simulink model "MPC_Shell3x3"  (R2021a)
settings: Solver=FixedStepAuto  StartTime=0  StopTime=1999  FixedStep=Ts  RelTol=1e-3
undefined symbols (not defined in the file or in its folder): L, R
libraries: simulink x3, mpclib x1, cstblocks x1
settings Model: Creator=Sergio Castaño  LastModifiedBy=Sergio
settings SolverCC: AlgebraicLoopSolver=TrustRegion
settings DataIOCC: LimitDataPoints=on  ReturnWorkspaceOutputs=off
settings OptimizationCC: DefaultParameterBehavior=Inlined  UseFloatMulNetSlope=on  InlineInvariantSignals=on  EnhancedBackFolding=on  PassReuseOutputArgsAs=Individual arguments  EfficientFloat2IntCast=on  LifeSpan=inf  EfficientTunableParamExpr=on
settings DebuggingCC: ParameterTunabilityLossMsg=error  AllowSymbolicDim=off  SFUnexpectedBacktrackingDiag=warning  SFNoUnconditionalDefaultTransitionDiag=warning  SFExecutionAtInitializationDiag=none  SFMachineParentedDataDiag=warning  ArithmeticOperatorsInVariantConditions=warning
settings HardwareCC: ProdBitPerSizeT=32  ProdBitPerPtrDiffT=32  ProdWordSize=32  ProdHWDeviceType=Specified
settings ModelReferenceCC: UpdateModelReferenceTargets=AssumeUpToDate  CheckModelReferenceTargetMessage=none  EnableParallelModelReferenceBuilds=on  PropagateSignalLabelsOutOfModel=off
settings SFSimCC: SimUseLocalCustomCode=off  MATLABDynamicMemAlloc=off  CustomCodeUndefinedFunction=UseInterfaceOnly
settings RTWCC: SystemTargetFile=ert.tlc  TemplateMakefile=ert_default_tmf  GenerateReport=on  RTWUseLocalCustomCode=off  IncludeHyperlinkInReport=on  LaunchReport=on  GenerateTraceInfo=on  GenerateTraceReport=on  GenerateTraceReportSl=on  GenerateTraceReportSf=on  GenerateTraceReportEml=on
settings CodeAppCC: ForceParamTrailComments=on  IgnoreCustomStorageClasses=off  OperatorAnnotations=on  SimulinkDataObjDesc=on  SFDataObjDesc=on  InsertBlockDesc=on  StateflowObjectComments=on
settings ERTTargetCC: GenerateSampleERTMain=on  SupportContinuousTime=on  InlinedParameterPlacement=NonHierarchical  ERTCustomFileTemplate=example_file_process.tlc
settings ConfigComp: CovMetricSettings=dw  CovSaveCumulativeToWorkspaceVar=on  CovSaveSingleToWorkspaceVar=on  CovExternalEMLEnable=off

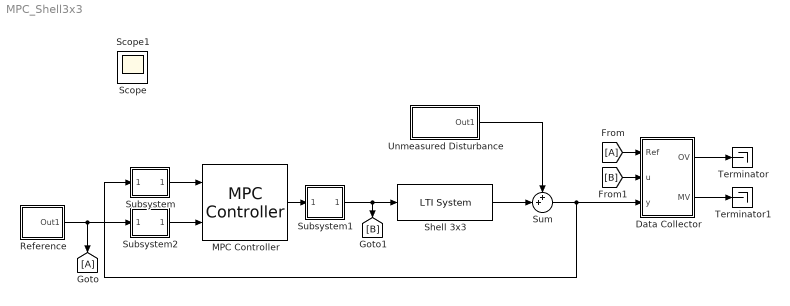
== system MPC_Shell3x3 ==
  Data Collector : Subsystem
  "MPC Controller " : mpclib/MPC Controller  SCDEnableBlockLinearizationSpecification=on  mpcobj=mpc_toolbox  is_multiple=0  enable_value=0  return_u0=off  updateMPCinCallerWorkspace=on  md_inport=off  mv_inport=off  uref_inport=off  return_cost=off  return_mvseq=off  return_qpstatus=off  return_xseq=off  return_state=off  return_ovseq=off  state_inport=off  umin_inport=off  umax_inport=off  ymin_inport=off  ymax_inport=off  cc_inport=off  ywt_inport=off  uwt_inport=off  duwt_inport=off  rhoeps_inport=off  pm_inport=off  MaximumP=10  HorizonChoice=FixedHorizon  n_ts=4  n_p=24  n_mv=3  n_md=0  n_ud=0  n_mo=3  n_uo=0  BlockDataType=double  SampleTimeInherited=off  switch_inport=off
  Reference : Subsystem
  Shell 3x3 : cstblocks/LTI System  sys=Psr  IC=[]
  Subsystem : Subsystem
  Subsystem1 : Subsystem
  Subsystem2 : Subsystem
  Sum : Sum  Inputs=++|
  Terminator : Terminator
  Terminator1 : Terminator
  Unmeasured Disturbance : Subsystem
  Scope : Scope
  Scope1 : Scope
  wires:
  "MPC Controller "/1 -> Subsystem1/1(In1)
  Shell 3x3/1 -> Sum/2
  Sum/1 -> Data Collector/3(y), Subsystem/1(In1)
  Subsystem/1(Out1) -> "MPC Controller "/1
  Subsystem2/1(Out1) -> "MPC Controller "/2
  Subsystem1/1(Out1) -> [B], Shell 3x3/1
  Reference/1(Out1) -> [A], Subsystem2/1(In1)
  Unmeasured Disturbance/1(Out1) -> Sum/1
  [A] -> Data Collector/1(Ref)
  [B] -> Data Collector/2(u)
  Data Collector/1(OV) -> Terminator/1
  Data Collector/2(MV) -> Terminator1/1

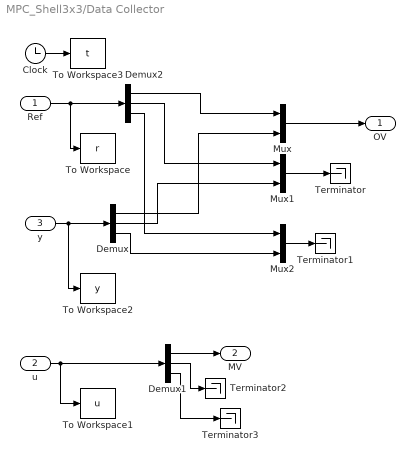
== system MPC_Shell3x3/Data Collector ==
  Ref : Inport
  u : Inport  Port=2
  y : Inport  Port=3
  Clock : Clock
  Demux : Demux  Outputs=3
  Demux1 : Demux  Outputs=3
  Demux2 : Demux  Outputs=3
  Mux : Mux  Inputs=2
  Mux1 : Mux  Inputs=2
  Mux2 : Mux  Inputs=2
  Terminator{,1..3} (4 alike) : Terminator
  To Workspace : ToWorkspace  VariableName=r  SampleTime=-1
  To Workspace1 : ToWorkspace  VariableName=u  SampleTime=-1
  To Workspace2 : ToWorkspace  VariableName=y  SampleTime=-1
  To Workspace3 : ToWorkspace  VariableName=t  SampleTime=-1
  OV : Outport
  MV : Outport  Port=2
  wires:
  y/1 -> To Workspace2/1, Demux/1
  u/1 -> Demux1/1, To Workspace1/1
  Ref/1 -> To Workspace/1, Demux2/1
  Demux2/1 -> Mux/1
  Demux/1 -> Mux/2
  Demux2/2 -> Mux1/1
  Demux/2 -> Mux1/2
  Demux2/3 -> Mux2/1
  Demux/3 -> Mux2/2
  Mux/1 -> OV/1
  Mux1/1 -> Terminator/1
  Mux2/1 -> Terminator1/1
  Demux1/1 -> MV/1
  Demux1/2 -> Terminator2/1
  Demux1/3 -> Terminator3/1
  Clock/1 -> To Workspace3/1

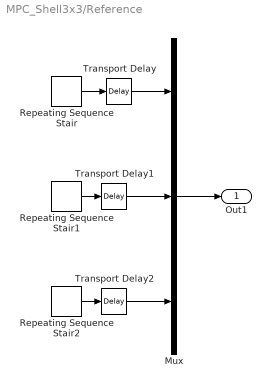
== system MPC_Shell3x3/Reference ==
  Mux : Mux  Inputs=3
  Repeating Sequence Stair : simulink/Sources/Repeating Sequence Stair  OutValues=[0.2 0 0.1 0.1 0].'  tsamp=400  OutMin=[]  OutMax=[]  OutDataTypeStr=double  OutputDataTypeScalingMode=double  OutDataType=fixdt(0,8)  ConRadixGroup=Best Precision: Vector-wise  OutScaling=2^-12
  Repeating Sequence Stair1 : simulink/Sources/Repeating Sequence Stair  OutValues=[0.2 0.4 0.3 0.3 0].'  tsamp=400  OutMin=[]  OutMax=[]  OutDataTypeStr=double  OutputDataTypeScalingMode=double  OutDataType=fixdt(0,8)  ConRadixGroup=Best Precision: Vector-wise  OutScaling=2^-12
  Repeating Sequence Stair2 : simulink/Sources/Repeating Sequence Stair  OutValues=[0.2 0.1 0 0 0].'  tsamp=400  OutMin=[]  OutMax=[]  OutDataTypeStr=double  OutputDataTypeScalingMode=double  OutDataType=fixdt(0,8)  ConRadixGroup=Best Precision: Vector-wise  OutScaling=2^-12
  Transport Delay : TransportDelay  DelayTime=40
  Transport Delay1 : TransportDelay  DelayTime=40
  Transport Delay2 : TransportDelay  DelayTime=40
  Out1 : Outport  VectorParamsAs1DForOutWhenUnconnected=off
  wires:
  Mux/1 -> Out1/1
  Repeating Sequence Stair/1 -> Transport Delay/1
  Repeating Sequence Stair1/1 -> Transport Delay1/1
  Repeating Sequence Stair2/1 -> Transport Delay2/1
  Transport Delay/1 -> Mux/1
  Transport Delay1/1 -> Mux/2
  Transport Delay2/1 -> Mux/3

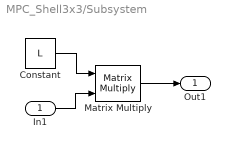
== system MPC_Shell3x3/Subsystem ==
  In1 : Inport
  Constant : Constant  Value=L
  Matrix Multiply : Product  Multiplication=Matrix(*)
  Out1 : Outport
  wires:
  Matrix Multiply/1 -> Out1/1
  In1/1 -> Matrix Multiply/2
  Constant/1 -> Matrix Multiply/1

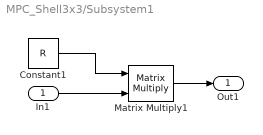
== system MPC_Shell3x3/Subsystem1 ==
  In1 : Inport
  Constant1 : Constant  Value=R
  Matrix Multiply1 : Product  Multiplication=Matrix(*)
  Out1 : Outport
  wires:
  Matrix Multiply1/1 -> Out1/1
  In1/1 -> Matrix Multiply1/2
  Constant1/1 -> Matrix Multiply1/1

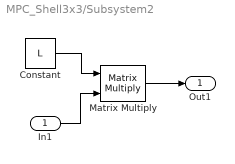
== system MPC_Shell3x3/Subsystem2 ==
  In1 : Inport
  Constant : Constant  Value=L
  Matrix Multiply : Product  Multiplication=Matrix(*)
  Out1 : Outport
  wires:
  Matrix Multiply/1 -> Out1/1
  Constant/1 -> Matrix Multiply/1
  In1/1 -> Matrix Multiply/2

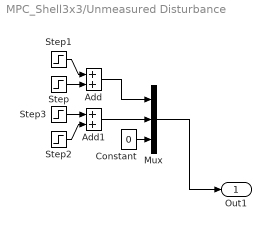
== system MPC_Shell3x3/Unmeasured Disturbance ==
  Add : Sum
  Add1 : Sum
  Constant : Constant  Value=0
  Mux : Mux  Inputs=3
  Step : Step  Time=1120  After=0.05  SampleTime=0
  Step1 : Step  Time=1100  After=-0.05  SampleTime=0
  Step2 : Step  Time=1420  After=-0.1  SampleTime=0
  Step3 : Step  Time=1400  After=0.1  SampleTime=0
  Out1 : Outport
  wires:
  Step2/1 -> Add1/2
  Add1/1 -> Mux/2
  Mux/1 -> Out1/1
  Constant/1 -> Mux/3
  Add/1 -> Mux/1
  Step1/1 -> Add/1
  Step/1 -> Add/2
  Step3/1 -> Add1/1
